simulink model "assignment_and_index"  (R2018b)
settings: Solver=VariableStepAuto  StartTime=0.0  StopTime=10.0  RelTol=1e-3
undefined symbols (not defined in the file or in its folder): A
settings Model: Creator=nishanthkumar.l  LastModifiedBy=nishanthkumar.l

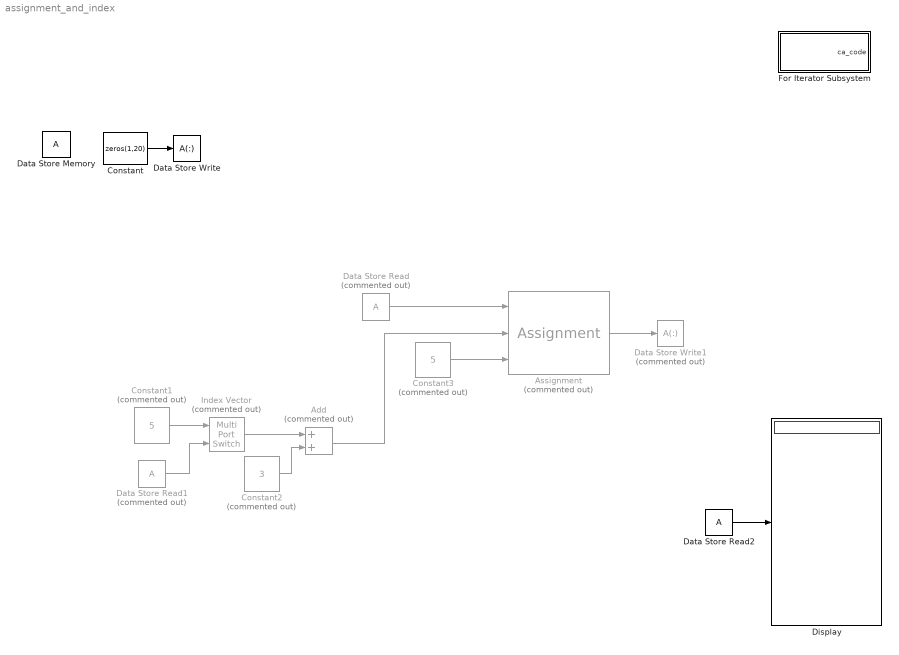
== system assignment_and_index ==
  Add : Sum  Commented=on
  Assignment : Assignment  Commented=on  DiagnosticForDimensions=Warning  IndexOptions=Index vector (port)  Indices=1  OutputSizes=1
  Constant : Constant  Priority=0  Value=zeros(1,20)  VectorParams1D=off  SampleTime=-1
  Constant1 : Constant  Commented=on  Value=5  VectorParams1D=off  SampleTime=-1
  Constant2 : Constant  Commented=on  Value=3  VectorParams1D=off  SampleTime=-1
  Constant3 : Constant  Commented=on  Value=5  VectorParams1D=off  SampleTime=-1
  Data Store Memory : DataStoreMemory  ReadBeforeWriteMsg=warning  WriteAfterWriteMsg=warning  WriteAfterReadMsg=warning  ShowAdditionalParam=off  Dimensions=[1 10]
  Data Store Read : DataStoreRead  Commented=on
  Data Store Read1 : DataStoreRead  Commented=on
  Data Store Read2 : DataStoreRead
  Data Store Write : DataStoreWrite  DataStoreElements=A(:)
  Data Store Write1 : DataStoreWrite  Commented=on  DataStoreElements=A(:)
  Display : Display
  For Iterator Subsystem : Subsystem  TreatAsAtomicUnit=on
  Index Vector : MultiPortSwitch  Commented=on  DataPortOrder=Zero-based contiguous  Inputs=1  zeroidx=on
  wires:
  Constant/1 -> Data Store Write/1
  Data Store Read1/1 -> Index Vector/2
  Constant1/1 -> Index Vector/1
  Index Vector/1 -> Add/1
  Constant2/1 -> Add/2
  Assignment/1 -> Data Store Write1/1
  Data Store Read/1 -> Assignment/1
  Add/1 -> Assignment/2
  Constant3/1 -> Assignment/3
  Data Store Read2/1 -> Display/1

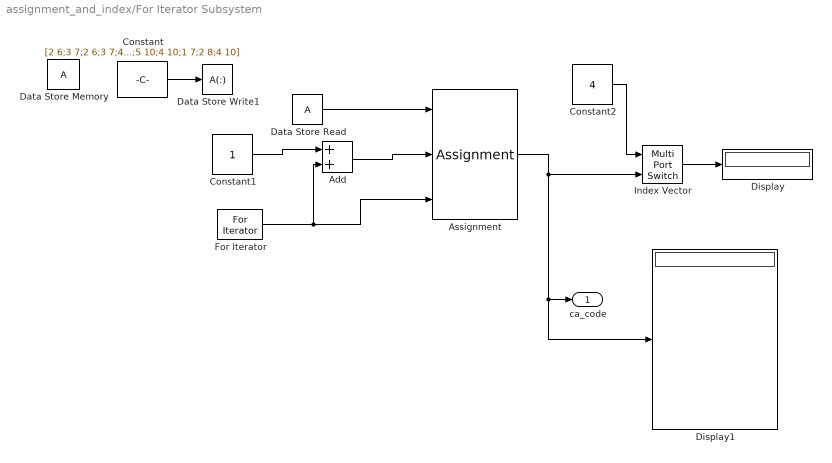
== system assignment_and_index/For Iterator Subsystem ==
  Add : Sum
  Assignment : Assignment  DiagnosticForDimensions=Warning  IndexOptions=Index vector (port)  Indices=[1:1023]  OutputSizes=1
  Constant : Constant  Priority=0  Value=[2 6;3 7;2 6;3 7;4 8;5 9;1 9;2 10;1 8;2 9;3 10;2 3;3 4;5 6;6 7;7 8;8 9;9 10;1 4;2 5;3 6;4 7;5 8;6 9;1 3;4 6;5 7;6 8;7 9;8 10;1 6;2 7;3 8;4 9;5 10;4 10;1 7;2 8;4 10]  VectorParams1D=off  SampleTime=-1
  Constant1 : Constant  VectorParams1D=off  SampleTime=-1
  Constant2 : Constant  Value=4  VectorParams1D=off  SampleTime=-1
  Data Store Memory : DataStoreMemory  ReadBeforeWriteMsg=warning  WriteAfterWriteMsg=warning  WriteAfterReadMsg=warning  ShowAdditionalParam=off  Dimensions=[1 5]
  Data Store Read : DataStoreRead
  Data Store Write1 : DataStoreWrite  DataStoreElements=A(:)
  Display : Display
  Display1 : Display
  For Iterator : ForIterator
  Index Vector : MultiPortSwitch  Inputs=1
  ca_code : Outport
  wires:
  For Iterator/1 -> Add/2, Assignment/3
  Data Store Read/1 -> Assignment/1
  Constant1/1 -> Add/1
  Add/1 -> Assignment/2
  Assignment/1 -> Index Vector/2, Display1/1, ca_code/1
  Constant2/1 -> Index Vector/1
  Index Vector/1 -> Display/1
  Constant/1 -> Data Store Write1/1
